simulink model "rtwdemo_sigobj_iv"  (Simulink 7.6)
settings: Solver=ode3  SolverMode=SingleTasking  StartTime=0.0  StopTime=20  FixedStep=1  RelTol=1e-3
PreLoadFcn:
  | rtwdemo_sigobj_iv_data
libraries: rtwdemowidgets x3
Description:
  | Controlling the Initial Value of Signals and States Using Signal Objects
settings Model: Creator=The MathWorks Inc.  CovMetricSettings=d  ExtModeTrigMode=oneshot  ExtModeArmWhenConnect=off  ExtModeAutoUpdateStatusClock=off  TunableVars=aa2  TunableVarsStorageClass=ExportedGlobal
settings MATStruct: SampleTime=1  Offset=0  Priority=[20.0]
settings DataIOCC: ExternalInput=[t u]  LimitDataPoints=off  SaveFormat=StructureWithTime  SaveOutput=off  SignalLogging=off  SaveTime=off  SignalLoggingName=sigsOut
settings OptimizationCC: InlineParams=on  InlineInvariantSignals=on  StateBitsets=on  DataBitsets=on  UseTempVars=on  EfficientFloat2IntCast=on  EfficientMapNaN2IntZero=off
settings DebuggingCC: ReadBeforeWriteMsg=EnableAllAsError  WriteAfterWriteMsg=EnableAllAsError  WriteAfterReadMsg=EnableAllAsError  CheckSSInitialOutputMsg=off  SolverPrmCheckMsg=none  SigSpecEnsureSampleTimeMsg=none  IntegerOverflowMsg=none  StrictBusMsg=ErrorOnBusTreatedAsVector
settings HardwareCC: ProdIntDivRoundTo=Zero  ProdEndianess=LittleEndian  ProdHWDeviceType=Generic->32-bit Embedded Processor  TargetHWDeviceType=Generic->32-bit Embedded Processor
settings RTWCC: TLCOptions=-aWarnNonSaturatedBlocks=0 -p0  GenerateReport=on  RTWVerbose=off  ProcessScript=grt_make_rtw_hook  LaunchReport=on
settings CodeAppCC: ForceParamTrailComments=on
settings GRTTargetCC: TargetFcnLib=ansi_tfl_tmw.mat

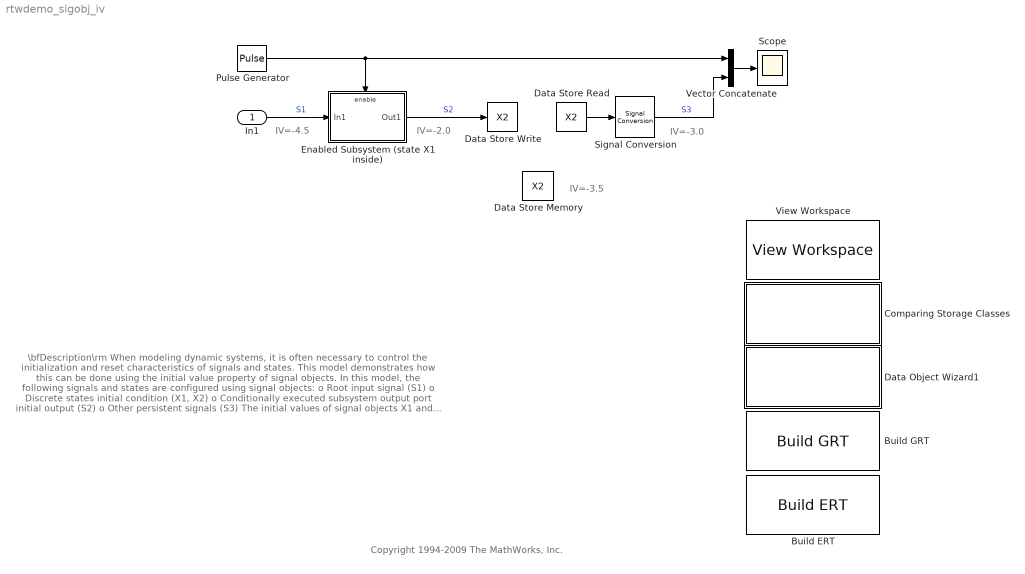
== system rtwdemo_sigobj_iv ==
  note: IV=-4.5
  note: IV=-3.5
  note: IV=-3.0
  note: IV=-2.0
  note: \bfDescription\rm
      | When modeling dynamic systems, it is often necessary to control the initialization and
      | reset characteristics of signals and states.  This model demonstrates how this can be
      | done using the initial value property of signal objects.
      |
      | In this model, the following signals and states are configured using signal objects:
      | o Root input signal (S1)
      | o Discrete states initial condition (X1, X2)
      | o Conditionally executed subsystem output port initial output (S2)
      | o Other persistent signals (S3)
      |
      | The initial values of signal objects X1 and S2 are specified using tunable parameters
      | aa1 and aa2 respectively.
      |
      | \bfInstructions\rm
      | 1. Simulate the model and inspect the results in the scope display.
      | 2. Generate code by double-clicking a blue button.  Inspect the generated code.
      | 3. Change the initial value of X1 or S2 (or the tunable parameters aa1 or aa2) in the
      |      Model Explorer and redo the simulation and code generation to inspect the results.
  note: Copyright 1994-2009 The MathWorks, Inc.
  In1 : Inport  OutDataTypeStr=double  PortDimensions=1  SampleTime=1
  Build ERT : rtwdemowidgets/Build ERT  SystemSampleTime=-1  attrib_overrides={}
  Build GRT : rtwdemowidgets/Build GRT  SystemSampleTime=-1  attrib_overrides={}
  Comparing Storage Classes : Subsystem
      settings: OpenFcn=edit rtwdemo_sigobj_iv_data.m
      mask Display: disp(['View M-file For\nCreating Variables\n(double-click)']);
  Data Object Wizard1 : Subsystem  Description=Signal object initial value
      settings: OpenFcn=helpview([docroot '/toolbox/rtw/helptargets.map'], 'sigobjiv')
      mask Type: Signal object initial value documentation
      mask Description: Signal object initial value documentation
      mask Display: disp('View User\nDocumentation\n(double-click)')
  Data Store Memory : DataStoreMemory  DataStoreName=X2  ReadBeforeWriteMsg=warning  WriteAfterWriteMsg=warning  WriteAfterReadMsg=warning  InitialValue=[]  StateMustResolveToSignalObject=on
  Data Store Read : DataStoreRead  DataStoreName=X2  SampleTime=1
  Data Store Write : DataStoreWrite  DataStoreName=X2
  Enabled Subsystem (state X1 inside) : Subsystem  TreatAsAtomicUnit=on
  Pulse Generator : DiscretePulseGenerator  PulseType=Time based  Period=10  PulseWidth=50  PhaseDelay=2
  Scope : Scope
  Signal Conversion : SignalConversion  ConversionOutput=Contiguous copy
  Vector Concatenate : Concatenate  Mode=Vector
  View Workspace : rtwdemowidgets/View Workspace  SystemSampleTime=-1
  wires:
  Pulse Generator/1 -> Enabled Subsystem (state X1 inside)/Enable, Vector Concatenate/1
  In1/1 -> Enabled Subsystem (state X1 inside)/1(In1)  "S1"
  Data Store Read/1 -> Signal Conversion/1
  Vector Concatenate/1 -> Scope/1
  Signal Conversion/1 -> Vector Concatenate/2  "S3"
  Enabled Subsystem (state X1 inside)/1(Out1) -> Data Store Write/1  "S2"

== system rtwdemo_sigobj_iv/Comparing Storage Classes ==

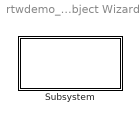
== system rtwdemo_sigobj_iv/Data Object Wizard1 ==
  Subsystem : Subsystem

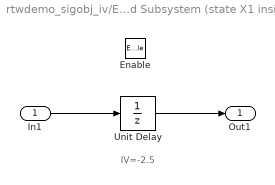
== system rtwdemo_sigobj_iv/Enabled Subsystem (state X1 inside) ==
  note: IV=-2.5
  In1 : Inport
  Enable : EnablePort  StatesWhenEnabling=reset
  Unit Delay : UnitDelay  X0=[]  StateIdentifier=X1  StateMustResolveToSignalObject=on
  Out1 : Outport  OutputWhenDisabled=reset
  wires:
  In1/1 -> Unit Delay/1
  Unit Delay/1 -> Out1/1

== system rtwdemo_sigobj_iv/Data Object Wizard1/Subsystem ==
